simulink model "QuadModelv"  (R2022a)
settings: Solver=ode4  StartTime=0.0  StopTime=inf  FixedStep=0.001  RelTol=1e-3
PreLoadFcn:
  | filepath  = fileparts(get_param(bdroot, 'FileName'));
  | cd(filepath);
InitFcn:
  | Init
values from neighbouring files (symbols this model uses):
  ModelFailEnable = 0    [Init.m]
  ModelInit_RPM = 0    [Init.m]
  ModelParam_BattHoverMinutes = 18    [Init.m]
  ModelParam_BattHoverThr = 0.609    [Init.m]
  ModelParam_envAltitude = -50    [Init.m]
  ModelParam_GPSEphFinal = 0.3    [Init.m]
  ModelParam_GPSEpvFinal = 0.4    [Init.m]
  ModelParam_GPSFix3DFix = 3    [Init.m]
  ModelParam_GPSSatsVisible = 10    [Init.m]
  ModelParam_motorCr = 842.1    [Init.m]
  ModelParam_motorJm = 0.0001287    [Init.m]
  ModelParam_motorMinThr = 0.05    [Init.m]
  ModelParam_motorT = 0.0214    [Init.m]
  ModelParam_motorWb = 22.83    [Init.m]
  ModelParam_noiseGPSSampTime = 0.2    [Init.m]
  ModelParam_noisePowerOffGainAccel = 0.04    [Init.m]
  ModelParam_noisePowerOffGainAccelZ = 0.03    [Init.m]
  ModelParam_noisePowerOffGainGyro = 0.02    [Init.m]
  ModelParam_noisePowerOffGainGyroZ = 0.025    [Init.m]
  ModelParam_noisePowerOffGainMag = 0.02    [Init.m]
  ModelParam_noisePowerOffGainMagZ = 0.035    [Init.m]
  ModelParam_noisePowerOnGainAccel = 0.8    [Init.m]
  ModelParam_noisePowerOnGainAccelZ = 4.5    [Init.m]
  ModelParam_noisePowerOnGainGyro = 2    [Init.m]
  ModelParam_noisePowerOnGainGyroZ = 1    [Init.m]
  ModelParam_noisePowerOnGainMag = 0.025    [Init.m]
  ModelParam_noisePowerOnGainMagZ = 0.05    [Init.m]
  ModelParam_rotorCm = 2.783e-07    [Init.m]
  ModelParam_rotorCt = 1.681e-05    [Init.m]
  ModelParam_uavCCm = [0.0035 0.0039 0.0034]    [Init.m]
  ModelParam_uavCd = 0.055    [Init.m]
  ModelParam_uavDearo = 0.12    [Init.m]
  ModelParam_uavJ = [ModelParam_uavJxx,0,0;0,ModelParam_uavJyy,0;0,0,ModelParam_uavJzz]    [Init.m]
  ModelParam_uavMass = 1.515    [Init.m]
  ModelParam_uavMotNumbs = int8(4)    [Init.m]
  ModelParam_uavR = 0.225    [Init.m]
  ModelParam_uavType = int8(3)    [Init.m]
undefined symbols (not defined in the file or in its folder): d_i, Earth, h_i, ModelParam_GPSEpvInitial, ModelParam_GPSEpvTimeConstant, Newton, Raphson, WGS84
libraries: simulink x9, QuadModelLib x7, sharedtransform x3, aerolibtransform2 x2, sharedutil x2, aerolibutil x2, aerolibasang x2, shared6dof x1, aerolibatmos2 x1, aerolibconvert2 x1, aerolibobsolete x1
(part 3 of 3)

== matlab function QuadModelv/Force and Moment Model/Ground Model ==
  settings: updateMethod=DISCRETE
  data: mg input; wb input; Xe input; F1 output; Ve input; M1 output; Quet input; terrainZ input; landed output; takeoff output
function [F1,M1,landed,takeoff] = fcn(mg,wb,Xe,Ve,Quet,terrainZ)
% This is a ground model that can provides reaction force and reaction torque

% persistent z0;
% if isempty(z0)
%      z0=0;
% end

persistent takeoffFlag;
if isempty(takeoffFlag)
     takeoffFlag=int8(0);
end

persistent landFlag;
if isempty(landFlag)
     landFlag=int8(1);
end

z=Xe(3)-terrainZ;

if (z<-0.3)&&(Ve(3)<-0.1)&&(takeoffFlag<0.5)
    takeoffFlag=int8(1);
    landFlag=int8(0);
end

if (z>-0.05)&&(Ve(3)>0.1)&&(landFlag<0.5)
    landFlag=int8(1);
    takeoffFlag=int8(0);
end

takeoff = takeoffFlag;
landed = landFlag;


F1=[0;0;0];
M1=[0;0;0];

if z>=0
%     if z>=0.3
%         if Ve(3)>=5
%             F1(3)=-mg(3)-1000*Ve(3);
%         else
%             F1(3)=-mg(3)-500*z-100*Ve(3);  
%         end
%     elseif z>=0.1
%         if Ve(3)>=2
%             F1(3)=-mg(3)-100*Ve(3);
%         else
%             F1(3)=-mg(3)-50*z-100*Ve(3);  
%         end
%     else
%          if Ve(3)>=1
%             F1(3)=-mg(3)-50*Ve(3);
%         else
%             F1(3)=-mg(3)-5*z-50*Ve(3);  
%         end       
%     end
    if z<0.05
        F1(3)=-mg(3)-10*Ve(3); 
    elseif z<0.1
        F1(3)=-mg(3)-0.5*z-20*Ve(3); 
    else
        F1(3)=-mg(3)-1*z-50*Ve(3); 
    end

    F1(1)=-50*Ve(1);
    F1(2)=-50*Ve(2);
    
%     if ~(isnan(Quet(2))||isnan(Quet(3))||isnan(Quet(4)))
%         M1=-200*[Quet(2);Quet(3);Quet(4)]-10*wb;
%     end
    
    M1=-20*[Quet(2);Quet(3);Quet(4)]-5*wb;
    M1 = M1 * abs(mg(3))*0.0333;
end

== matlab function QuadModelv/Battery FaultModel/MATLAB Function ==
  data: load input; time input; EffRatio output; hover_time input; hover_thr input; motorNumbs input; cell_voltage output; isUseCustomHovTime input; CustomHovTime input; isPowOff input; isLowVoltage input; remainVoltageRatio input; islowCapacity input; remainCapacityRatio input; remCapacity output
function [EffRatio, cell_voltage,remCapacity]= LiPo(load,time,hover_time,hover_thr,motorNumbs,isUseCustomHovTime,CustomHovTime,isPowOff,isLowVoltage,remainVoltageRatio,islowCapacity,remainCapacityRatio)
%% battery model
%================================Constants=================================

delta_t = 0.01;
%max_current = 5.500;                % maximum current per motor             (A)
%aux_current = 0.100;                % current of auxillary components       (A)        
%capacity = 1.000;                   % LiPo current capacity                 (Ah)                                 
%cells = 2;                          % LiPo cell count

%==========================================================================

persistent discharge;
if isempty(discharge)
    discharge = 0;
end

persistent startTime;
if isempty(startTime)
    startTime = 0;
end

persistent reset;
if isempty(reset)
    reset = 0;
end

discharge_capacity=0;

% 低电量故障
if islowCapacity
   hover_time = hover_time*remainCapacityRatio(1);
   isUseCustomHovTime=false;
end


if ~isUseCustomHovTime 
    capacity=1;
    
    if hover_time<0.01
        hover_time=0.01;
    end
    
    hover_current=1/(hover_time*1.4/60);
    current=0;
    for i=1:motorNumbs
        current=current+hover_current*(load(i)/hover_thr)^2;
    end
    aux_current=0.5;
    %current = sum(hover_current .* (load/hover_thr).^2) + aux_current;
    current =(current+aux_current)/double(motorNumbs);
    discharge = current * (delta_t / 3600) + discharge;
    discharge_capacity = discharge / capacity;    
end




%如果启用电池模型且使用自定义续航时间
if isUseCustomHovTime
      hover_time=CustomHovTime(1)*1.4*60;
      if reset<0.5
         startTime=time;
         reset=1;
      end
      if hover_time<0.01
          hover_time=0.01;
      end
     discharge_capacity=(time-startTime)/hover_time;
else
    %使用默认的续航算法
    reset=0;
end


if discharge_capacity<0
    discharge_capacity=0;
end
if discharge_capacity>1
    discharge_capacity=1;
end


%电量与电压的曲线
if (0 <= discharge_capacity) && (discharge_capacity <=0.20)
    cell_voltage = -14.029*discharge_capacity^3 + 16.975*discharge_capacity^2 - 5.3339*discharge_capacity + 4.2;
elseif (0.20 < discharge_capacity) && (discharge_capacity < 0.70)
    cell_voltage = -0.2*discharge_capacity + 3.74;
else
    cell_voltage = -48*discharge_capacity^3 + 89.6*discharge_capacity^2 - 55.08*discharge_capacity + 14.716;
end

if cell_voltage < 0.5
    cell_voltage = 0;
end

% 电池失效故障
if isPowOff
     cell_voltage = 0; 
end

% 低电压故障
if isLowVoltage
    if remainVoltageRatio(1)>1
        remainVoltageRatio(1)=1;
    elseif remainVoltageRatio(1)<0
        remainVoltageRatio(1)=0;
    end
     cell_voltage = remainVoltageRatio(1)*4.2;
end


%如果电池模型未启用，续航为无穷久，同时各个全局变量归零
if ~isUseCustomHovTime&&~isPowOff&&~isLowVoltage&&~islowCapacity
    cell_voltage=4.2;
    discharge = 0;
    startTime = 0;
    reset = 0;
end

%效率矩阵
EffRatio=cell_voltage/4.2;
remCapacity=1-discharge_capacity;
%==========================================================================

== matlab function QuadModelv/LogSelectModel/MATLAB Function ==
  data: FaultIDs input; y output; D123450 input; D123451 input; D123452 input; unused input; unused90 input; unused91 input; D123456 input; unused92 input; unused93 input; D123459 input; unused94 input; unused95 input; unused96 input; unused97 input; D123544 input; D123545 input; D123546 input; D123547 input; D123548 input
function y = fcn(FaultIDs,D123450,D123451,D123452,~,~,~,D123456,~,~,D123459,~,~,~,~,D123544,D123545,D123546,D123547,D123548)

y = zeros(23,1);

FaultNum = 0;
for i = 1:8
    if FaultIDs(i)~=0
        FaultNum = FaultNum + 1;
    end
end


if FaultNum == 1
    if FaultIDs(1) == 123450|| FaultIDs(1) == 123549
        for i = 1:8
            y(i) = D123450(i);
        end
    elseif FaultIDs(1) == 123451
        for i = 1:8
            y(i) = D123451(i);
        end
    elseif FaultIDs(1) == 123452 || FaultIDs(1) == 123453 || FaultIDs(1) == 123454 || FaultIDs(1) == 123455
        for i = 1:2
            y(i) = D123452(i);
        end
    elseif FaultIDs(1) == 123456 || FaultIDs(1) == 123457 || FaultIDs(1) == 123458
        for i = 1:4
            y(i) = D123456(i);
        end
    elseif FaultIDs(1) == 123459 || FaultIDs(1) == 123540 || FaultIDs(1) == 123541 || FaultIDs(1) == 123542 || FaultIDs(1) == 123543
        for i = 1:6
            y(i) = D123459(i);
        end
    elseif FaultIDs(1) == 123544
        for i = 1:3
            y(i) = D123544(i);
        end
    elseif FaultIDs(1) == 123545
        for i = 1:3
            y(i) = D123545(i);
        end
    elseif FaultIDs(1) == 123546
        for i = 1:3
            y(i) = D123546(i);
        end
    elseif FaultIDs(1) == 123547
        y(1) = D123547(1);
    elseif FaultIDs(1) == 123548
        for i = 1:3
            y(i) = D123548(i);
        end
    end
end

if FaultNum == 2
    if FaultIDs(1) == 123450|| FaultIDs(1) == 123549
        for i = 1:8
            y(i) = D123450(i);
        end
        if FaultIDs(2) == 123451
            j = 1;
            for i = 9:16
                y(i) = D123451(j);
                j = j + 1;
            end
        elseif FaultIDs(2) == 123452 || FaultIDs(2) == 123453 || FaultIDs(2) == 123454 || FaultIDs(1) == 123455
            j = 1;
            for i = 9:10
                y(i) = D123452(j);
                j = j + 1;
            end
        elseif FaultIDs(2) == 123456 || FaultIDs(2) == 123457 || FaultIDs(2) == 123458
            j = 1;
            for i = 9:12
                y(i) = D123456(j);
                j = j + 1;
            end
        elseif FaultIDs(2) == 123459 || FaultIDs(2) == 123540 || FaultIDs(2) == 123541 || FaultIDs(2) == 123542 || FaultIDs(2) == 123543
            j = 1;
            for i = 9:14
                y(i) = D123459(j);
                j = j + 1;
            end
        elseif FaultIDs(2) == 123544
            j = 1;
            for i = 9:11
                y(i) = D123544(j);
                j = j + 1;
            end
        elseif FaultIDs(2) == 123545
            j = 1;
            for i = 9:11
                y(i) = D123545(j);
                j = j + 1;
            end
        elseif FaultIDs(2) == 123546
            j = 1;
            for i = 9:11
                y(i) = D123546(j);
                j = j + 1;
            end
        elseif FaultIDs(2) == 123547
            y(9) = D123547;
        elseif FaultIDs(2) == 123548
            j = 1;
            for i = 9:11
                y(i) = D123548(j);
                j = j + 1;
            end
        end
    elseif FaultIDs(1) == 123451
        for i = 1:8
            y(i) = D123451(i);
        end
        if FaultIDs(2) == 123450|| FaultIDs(2) == 123549
            j = 1;
            for i = 9:16
                y(i) = D123450(j);
                j = j + 1;
            end
        elseif FaultIDs(2) == 123452 || FaultIDs(2) == 123453 || FaultIDs(2) == 123454 || FaultIDs(1) == 123455
            j = 1;
            for i = 9:10
                y(i) = D123452(j);
                j = j + 1;
            end
        elseif FaultIDs(2) == 123456 || FaultIDs(2) == 123457 || FaultIDs(2) == 123458
            j = 1;
            for i = 9:12
                y(i) = D123456(j);
                j = j + 1;
            end
        elseif FaultIDs(2) == 123459 || FaultIDs(2) == 123540 || FaultIDs(2) == 123541 || FaultIDs(2) == 123542 || FaultIDs(2) == 123543
            j = 1;
            for i = 9:14
                y(i) = D123459(j);
                j = j + 1;
            end
        elseif FaultIDs(2) == 123544
            j = 1;
            for i = 9:11
                y(i) = D123544(j);
                j = j + 1;
            end
        elseif FaultIDs(2) == 123545
            j = 1;
            for i = 9:11
                y(i) = D123545(j);
                j = j + 1;
            end
        elseif FaultIDs(2) == 123546
            j = 1;
            for i = 9:11
                y(i) = D123546(j);
                j = j + 1;
            end
        elseif FaultIDs(2) == 123547
            y(9) = D123547;
        elseif FaultIDs(2) == 123548
            j = 1;
            for i = 9:11
                y(i) = D123548(j);
                j = j + 1;
            end
        end
    elseif FaultIDs(1) == 123452 || FaultIDs(1) == 123453 || FaultIDs(1) == 123454 || FaultIDs(1) == 123455
        for i = 1:2
            y(i) = D123452(i);
        end
        if FaultIDs(2) == 123450|| FaultIDs(2) == 123549
            j = 1;
            for i = 3:10
                y(i) = D123450(j);
                j = j + 1;
            end
        elseif FaultIDs(2) == 123451
            j = 1;
            for i = 3:10
                y(i) = D123451(j);
                j = j + 1;
            end
        elseif FaultIDs(2) == 123456 || FaultIDs(2) == 123457 || FaultIDs(2) == 123458
            j = 1;
            for i = 3:6
                y(i) = D123456(j);
                j = j + 1;
            end
        elseif FaultIDs(2) == 123459 || FaultIDs(2) == 123540 || FaultIDs(2) == 123541 || FaultIDs(2) == 123542 || FaultIDs(2) == 123543
            j = 1;
            for i = 3:8
                y(i) = D123459(j);
                j = j + 1;
            end
        elseif FaultIDs(2) == 123544
            j = 1;
            for i = 3:5
                y(i) = D123544(j);
                j = j + 1;
            end
        elseif FaultIDs(2) == 123545
            j = 1;
            for i = 3:5
                y(i) = D123545(j);
                j = j + 1;
            end
        elseif FaultIDs(2) == 123546
            j  = 1;
            for i = 3:5
                y(i) = D123546(j);
                j = j + 1;
            end
        elseif FaultIDs(2) == 123547
            y(3) = D123547;
        elseif FaultIDs(2) == 123548
            j = 1;
            for i = 3:5
                y(i) = D123548(j);
                j = j + 1;
            end
        end
    elseif FaultIDs(1) == 123456 || FaultIDs(1) == 123457 || FaultIDs(1) == 123458
        for i = 1:4
            y(i) = D123456(i);
        end
        if FaultIDs(2) == 123450|| FaultIDs(2) == 123549
            j = 1;
            for i = 5:12
                y(i) = D123450(j);
                j = j + 1;
            end
        elseif FaultIDs(2) == 123451
            j = 1;
            for i = 5:12
                y(i) = D123451(j);
                j = j + 1;
            end
        elseif FaultIDs(2) == 123452 || FaultIDs(2) == 123453 || FaultIDs(2) == 123454 || FaultIDs(2) == 123455
            j = 1;
            for i = 5:6
                y(i) = D123452(j);
                j = j + 1;
            end
        elseif FaultIDs(2) == 123459 || FaultIDs(2) == 123540 || FaultIDs(2) == 123541 || FaultIDs(2) == 123542 || FaultIDs(2) == 123543
            j = 1;
            for i = 5:10
                y(i) = D123459(j);
                j = j + 1;
            end
        elseif FaultIDs(2) == 123544
            j = 1;
            for i = 5:7
                y(i) = D123544(j);
                j = j + 1;
            end
        elseif FaultIDs(2) == 123545
            j = 1;
            for i = 5:7
                y(i) = D123545(j);
                j = j + 1;
            end
        elseif FaultIDs(2) == 123546
            j = 1;
            for i = 5:7
                y(i) = D123546(j);
                j = j + 1;
            end
        elseif FaultIDs(2) == 123547
            y(5) = D123547;
        elseif FaultIDs(2) == 123548
            j = 1;
            for i = 5:7
                y(i) = D123548(j);
                j = j + 1;
            end
        end
    elseif FaultIDs(1) == 123459 || FaultIDs(1) == 123540 || FaultIDs(1) == 123541 || FaultIDs(1) == 123542 || FaultIDs(1) == 123543
        for i = 1:6
            y(i) = D123459(i);
        end
        if FaultIDs(2) == 123450|| FaultIDs(2) == 123549
            j = 1;
            for i = 7:14
                y(i) = D123450(j);
                j = j + 1;
            end
        elseif FaultIDs(2) == 123451
            j = 1;
            for i = 7:14
                y(i) = D123451(j);
                j = j + 1;
            end
        elseif FaultIDs(2) == 123452 || FaultIDs(2) == 123453 || FaultIDs(2) == 123454 || FaultIDs(2) == 123455
            j = 1;
            for i = 7:8
                y(i) = D123452(j);
                j = j + 1;
            end
        elseif FaultIDs(2) == 123456 || FaultIDs(2) == 123457 || FaultIDs(2) == 123458
            j = 1;
            for i = 7:12
                y(i) = D123456(j);
                j = j + 1;
            end
        elseif FaultIDs(2) == 123544
            j = 1;
            for i = 7:9
                y(i) = D123544(j);
                j = j + 1;
            end
        elseif FaultIDs(2) == 123545
            j = 1;
            for i = 7:9
                y(i) = D123545(j);
                j = j + 1;
            end
        elseif FaultIDs(2) == 123546
            j = 1;
            for i = 7:9
                y(i) = D123546(j);
                j = j + 1;
            end
        elseif FaultIDs(2) == 123547
            y(7) = D123547;
        elseif FaultIDs(2) == 123548
            j = 1;
            for i = 7:9
                y(i) = D123548(j);
                j = j + 1;
            end
        end
    elseif FaultIDs(1) == 123544
        for i = 1:3
            y(i) = D123544(i);
        end
        if FaultIDs(2) == 123450|| FaultIDs(2) == 123549
            j = 1;
            for i = 4:11
                y(i) = D123450(j);
                j = j + 1;
            end
        elseif FaultIDs(2) == 123451
            j = 1;
            for i = 4:11
                y(i) = D123451(j);
                j = j + 1;
            end
        elseif FaultIDs(2) == 123452 || FaultIDs(2) == 123453 || FaultIDs(2) == 123454 || FaultIDs(2) == 123455
            j = 1;
            for i = 4:5
                y(i) = D123452(j);
                j = j + 1;
            end
        elseif FaultIDs(2) == 123456 || FaultIDs(2) == 123457 || FaultIDs(2) == 123458
            j = 1;
            for i = 4:9
                y(i) = D123456(j);
                j = j + 1;
            end
        elseif FaultIDs(2) == 123459 || FaultIDs(2) == 123540 || FaultIDs(2) == 123541 || FaultIDs(2) == 123542 || FaultIDs(2) == 123543
            j = 1;
            for i = 4:9
                y(i) = D123459(j);
                j = j + 1;
            end
        elseif FaultIDs(2) == 123545
            j = 1;
            for i = 4:6
                y(i) = D123545(j);
                j = j + 1;
            end
        elseif FaultIDs(2) == 123546
            j = 1;
            for i = 4:6
                y(i) = D123546(j);
                j = j + 1;
            end
        elseif FaultIDs(2) == 123547
            y(4) = D123547;
        elseif FaultIDs(2) == 123548
            j = 1;
            for i = 4:6
                y(i) = D123548(j);
                j = j + 1;
            end
        end
    elseif FaultIDs(1) == 123545
        for i = 1:3
            y(i) = D123545(i);
        end
        if FaultIDs(2) == 123450|| FaultIDs(2) == 123549
            j = 1;
            for i = 4:11
                y(i) = D123450(j);
                j = j + 1;
            end
        elseif FaultIDs(2) == 123451
            j = 1;
            for i = 4:11
                y(i) = D123451(j);
                j = j + 1;
            end
        elseif FaultIDs(2) == 123452 || FaultIDs(2) == 123453 || FaultIDs(2) == 123454 || FaultIDs(2) == 123455
            j = 1;
            for i = 4:5
                y(i) = D123452(j);
                j = j + 1;
            end
        elseif FaultIDs(2) == 123456 || FaultIDs(2) == 123457 || FaultIDs(2) == 123458
            j = 1;
            for i = 4:9
                y(i) = D123456(j);
                j = j + 1;
            end
        elseif FaultIDs(2) == 123459 || FaultIDs(2) == 123540 || FaultIDs(2) == 123541 || FaultIDs(2) == 123542 || FaultIDs(2) == 123543
            j = 1;
            for i = 4:9
                y(i) = D123459(j);
                j = j + 1;
            end
        elseif FaultIDs(2) == 123544
            j = 1;
            for i = 4:6
                y(i) = D123544(j);
                j = j + 1;
            end
        elseif FaultIDs(2) == 123546
            j = 1;
            for i = 4:6
                y(i) = D123546(j);
                j = j + 1;
            end
        elseif FaultIDs(2) == 123547
            y(4) = D123547;
        elseif FaultIDs(2) == 123548
            j = 1;
            for i = 4:6
                y(i) = D123548(j);
                j = j + 1;
            end
        end
    elseif FaultIDs(1) == 123546
        for i = 1:3
            y(i) = D123545(i);
        end
        if FaultIDs(2) == 123450|| FaultIDs(2) == 123549
            j = 1;
            for i = 4:11
                y(i) = D123450(j);
                j = j + 1;
            end
        elseif FaultIDs(2) == 123451
            j = 1;
            for i = 4:11
                y(i) = D123451(j);
                j = j + 1;
            end
        elseif FaultIDs(2) == 123452 || FaultIDs(2) == 123453 || FaultIDs(2) == 123454 || FaultIDs(2) == 123455
            j = 1;
            for i = 4:5
                y(i) = D123452(j);
                j = j + 1;
            end
        elseif FaultIDs(2) == 123456 || FaultIDs(2) == 123457 || FaultIDs(2) == 123458
            j = 1;
            for i = 4:9
                y(i) = D123456(j);
                j = j + 1;
            end
        elseif FaultIDs(2) == 123459 || FaultIDs(2) == 123540 || FaultIDs(2) == 123541 || FaultIDs(2) == 123542 || FaultIDs(2) == 123543
            j = 1;
            for i = 4:9
                y(i) = D123459(j);
                j = j + 1;
            end
        elseif FaultIDs(2) == 123544
            j = 1;
            for i = 4:6
                y(i) = D123544(j);
                j = j + 1;
            end
        elseif FaultIDs(2) == 123545
            j = 1;
            for i = 4:6
                y(i) = D123545(j);
                j = j + 1;
            end
        elseif FaultIDs(2) == 123547
            y(4) = D123547;
        elseif FaultIDs(2) == 123548
            j = 1;
            for i = 4:6
                y(i) = D123548(j);
                j = j + 1;
            end
        end
    elseif FaultIDs(1) == 123547
        y(1) = D123547(1);
        if FaultIDs(2) == 123450|| FaultIDs(2) == 123549
            j = 1;
            for i = 2:9
                y(i) = D123450(j);
                j = j + 1;
            end
        elseif FaultIDs(2) == 123451
            j = 1;
            for i = 2:9
                y(i) = D123451(j);
                j = j + 1;
            end
        elseif FaultIDs(2) == 123452 || FaultIDs(2) == 123453 || FaultIDs(2) == 123454 || FaultIDs(2) == 123455
            j = 1;
            for i = 2:3
                y(i) = D123452(j);
                j = j + 1;
            end
        elseif FaultIDs(2) == 123456 || FaultIDs(2) == 123457 || FaultIDs(2) == 123458
            j = 1;
            for i = 2:7
                y(i) = D123456(j);
                j = j + 1;
            end
        elseif FaultIDs(2) == 123459 || FaultIDs(2) == 123540 || FaultIDs(2) == 123541 || FaultIDs(2) == 123542 || FaultIDs(2) == 123543
            j = 1;
            for i = 2:7
                y(i) = D123459(j);
                j = j + 1;
            end
        elseif FaultIDs(2) == 123544
            j = 1;
            for i = 2:4
                y(i) = D123544(j);
                j = j + 1;
            end
        elseif FaultIDs(2) == 123545
            j = 1;
            for i = 2:4
                y(i) = D123545(j);
                j = j + 1;
            end
        elseif FaultIDs(2) == 123546
            j = 1;
           for i = 2:4
                y(i) = D123546(j);
                j = j + 1;
            end
        elseif FaultIDs(2) == 123548
            j = 1;
            for i = 2:4
                y(i) = D123548(j);
                j = j + 1;
            end
        end
    elseif FaultIDs(1) == 123548
        for i = 1:3
            y(i) = D123548(i);
        end
        if FaultIDs(2) == 123450|| FaultIDs(2) == 123549
            j = 1;
            for i = 4:11
                y(i) = D123450(j);
                j = j + 1;
            end
        elseif FaultIDs(2) == 123451
            j = 1;
            for i = 4:11
                y(i) = D123451(j);
                j = j + 1;
            end
        elseif FaultIDs(2) == 123452 || FaultIDs(2) == 123453 || FaultIDs(2) == 123454 || FaultIDs(2) == 123455
            j = 1;
            for i = 4:5
                y(i) = D123452(j);
                j = j + 1;
            end
        elseif FaultIDs(2) == 123456 || FaultIDs(2) == 123457 || FaultIDs(2) == 123458
            j = 1;
            for i = 4:9
                y(i) = D123456(j);
                j = j + 1;
            end
        elseif FaultIDs(2) == 123459 || FaultIDs(2) == 123540 || FaultIDs(2) == 123541 || FaultIDs(2) == 123542 || FaultIDs(2) == 123543
            j = 1;
            for i = 4:9
                y(i) = D123459(j);
                j = j + 1;
            end
        elseif FaultIDs(2) == 123544
            j = 1;
            for i = 4:6
                y(i) = D123544(j);
                j = j + 1;
            end
        elseif FaultIDs(2) == 123545
            j = 1;
            for i = 4:6
                y(i) = D123545(j);
                j = j + 1;
            end
        elseif FaultIDs(2) == 123547
            y(4) = D123547;
        elseif FaultIDs(2) == 123546
            j = 1;
            for i = 4:6
                y(i) = D123546(j);
                j = j + 1;
            end
        end
    end
end

if FaultNum >= 3
    if any(find(FaultIDs==123450|FaultIDs==123549))&&any(find(FaultIDs==123452|FaultIDs==123453|FaultIDs==123454|FaultIDs==123455))&&any(find(FaultIDs==123456|FaultIDs==123457|FaultIDs==123458))
        for i = 1:8
            y(i) = D123450(i);
        end
        j = 1;
        for i = 9:10
            y(i) = D123452(j);
            j = j + 1;
        end
        k = 1;
        for i = 11:14
            y(i) = D123456(k);
            k = k + 1;
        end
    elseif any(find(FaultIDs==123450|FaultIDs==123549))&&any(find(FaultIDs==123452|FaultIDs==123453|FaultIDs==123454|FaultIDs==123455))&&any(find(FaultIDs==123459|FaultIDs==123540|FaultIDs==123541|FaultIDs==123542|FaultIDs==123543))
        for i = 1:8
            y(i) = D123450(i);
        end
        j = 1;
        for i = 9:10
            y(i) = D123452(j);
            j = j + 1;
        end
        k = 1;
        for i = 11:16
            y(i) = D123459(k);
            k = k + 1;
        end
    elseif any(find(FaultIDs==123450|FaultIDs==123549))&&any(find(FaultIDs==123452|FaultIDs==123453|FaultIDs==123454|FaultIDs==123455))&&any(find(FaultIDs==123544|FaultIDs==123545|FaultIDs==123546|FaultIDs==123548|FaultIDs==123547))
        for i = 1:8
            y(i) = D123450(i);
        end
        j = 1;
        for i = 9:10
            y(i) = D123452(j);
            j = j + 1;
        end
        k = 1;
        if any(find(FaultIDs==123544))
            for i = 11:13
                y(i) = D123544(k);
                k = k + 1;
            end
        elseif any(find(FaultIDs==123545))
            for i = 11:13
                y(i) = D123545(k);
                k = k + 1;
            end
        elseif any(find(FaultIDs==123546))
            for i = 11:13
                y(i) = D123546(k);
                k = k + 1;
            end
        elseif any(find(FaultIDs==123548))
            for i = 11:13
                y(i) = D123548(k);
                k = k + 1;
            end
        elseif any(find(FaultIDs==123547))
           y(11) = D123547;
        end
    elseif any(find(FaultIDs==123452|FaultIDs==123453|FaultIDs==123454|FaultIDs==123455))&&any(find(FaultIDs==123456|FaultIDs==123457|FaultIDs==123458))&&any(find(FaultIDs==123459|FaultIDs==123540|FaultIDs==123541|FaultIDs==123542|FaultIDs==123543))
        for i = 1:2
            y(i) = D123452(i);
        end
        j = 1;
        for i = 3:6
            y(i) = D123456(j);
            j = j + 1;
        end
        k = 1;
        for i = 7:12
            y(i) = D123459(k);
            k = k + 1;
        end
    elseif any(find(FaultIDs==123452|FaultIDs==123453|FaultIDs==123454|FaultIDs==123455))&&any(find(FaultIDs==123456|FaultIDs==123457|FaultIDs==123458))&&any(find(FaultIDs==123544|FaultIDs==123545|FaultIDs==123546|FaultIDs==123548|FaultIDs==123547))
        for i = 1:2
            y(i) = D123452(i);
        end
        j = 1;
        for i = 3:6
            y(i) = D123456(j);
            j = j + 1;
        end
        k = 1;
        if any(find(FaultIDs==123544))
            for i = 7:9
                y(i) = D123544(k);
                k = k + 1;
            end
        elseif any(find(FaultIDs==123545))
            for i = 7:9
                y(i) = D123545(k);
                k = k + 1;
            end
        elseif any(find(FaultIDs==123546))
            for i = 7:9
                y(i) = D123546(k);
                k = k + 1;
            end
        elseif any(find(FaultIDs==123548))
            for i = 7:9
                y(i) = D123548(k);
                k = k + 1;
            end
        elseif any(find(FaultIDs==123547))
           y(7) = D123547;
        end
    elseif any(find(FaultIDs==123456|FaultIDs==123457|FaultIDs==123458))&&any(find(FaultIDs==123544|FaultIDs==123545|FaultIDs==123546|FaultIDs==123548|FaultIDs==123547))&&any(find(FaultIDs==123459|FaultIDs==123540|FaultIDs==123541|FaultIDs==123542|FaultIDs==123543))
        for i = 1:4
            y(i) = D123456(i);
        end
        j = 1;
        for i = 5:10
            y(i) = D123459(j);
            j = j + 1;
        end
        k = 1;
        if any(find(FaultIDs==123544))
            for i = 11:13
                y(i) = D123544(k);
                k = k + 1;
            end
        elseif any(find(FaultIDs==123545))
            for i = 11:13
                y(i) = D123545(k);
                k = k + 1;
            end
        elseif any(find(FaultIDs==123546))
            for i = 11:13
                y(i) = D123546(k);
                k = k + 1;
            end
        elseif any(find(FaultIDs==123548))
            for i = 11:13
                y(i) = D123548(k);
                k = k + 1;
            end
        elseif any(find(FaultIDs==123547))
           y(11) = D123547;
        end
    elseif any(find(FaultIDs==123450|FaultIDs==123549))&&any(find(FaultIDs==123456|FaultIDs==123457|FaultIDs==123458))&&any(find(FaultIDs==123459|FaultIDs==123540|FaultIDs==123541|FaultIDs==123542|FaultIDs==123543))
        for i = 1:8
            y(i) = D123450(i);
        end
        j = 1;
        for i = 9:12
            y(i) = D123456(j);
            j = j + 1;
        end
        k = 1;
        for i = 13:18
            y(i) = D123459(k);
            k = k + 1;
        end
    elseif any(find(FaultIDs==123450|FaultIDs==123549))&&any(find(FaultIDs==123456|FaultIDs==123457|FaultIDs==123458))&&any(find(FaultIDs==123544|FaultIDs==123545|FaultIDs==123546|FaultIDs==123548|FaultIDs==123547))
        for i = 1:8
            y(i) = D123450(i);
        end
        j = 1;
        for i = 9:12
            y(i) = D123456(j);
            j = j + 1;
        end
        k = 1;
        if any(find(FaultIDs==123544))
            for i = 13:15
                y(i) = D123544(k);
                k = k + 1;
            end
        elseif any(find(FaultIDs==123545))
            for i = 13:15
                y(i) = D123545(k);
                k = k + 1;
            end
        elseif any(find(FaultIDs==123546))
            for i = 13:15
                y(i) = D123546(k);
                k = k + 1;
            end
        elseif any(find(FaultIDs==123548))
            for i = 13:15
                y(i) = D123548(k);
                k = k + 1;
            end
        elseif any(find(FaultIDs==123547))
           y(13) = D123547;
        end
    elseif any(find(FaultIDs==123450|FaultIDs==123549))&&any(find(FaultIDs==123459|FaultIDs==123540|FaultIDs==123541|FaultIDs==123542|FaultIDs==123543))&&any(find(FaultIDs==123544|FaultIDs==123545|FaultIDs==123546|FaultIDs==123548|FaultIDs==123547))
        for i = 1:8
            y(i) = D123450(i);
        end
        j = 1;
        for i = 9:14
            y(i) = D123459(j);
            j = j + 1;
        end
        k = 1;
        if any(find(FaultIDs==123544))
            for i = 15:17
                y(i) = D123544(k);
                k = k + 1;
            end
        elseif any(find(FaultIDs==123545))
            for i = 15:17
                y(i) = D123545(k);
                k = k + 1;
            end
        elseif any(find(FaultIDs==123546))
            for i = 15:17
                y(i) = D123546(k);
                k = k + 1;
            end
        elseif any(find(FaultIDs==123548))
            for i = 15:17
                y(i) = D123548(k);
                k = k + 1;
            end
        elseif any(find(FaultIDs==123547))
           y(15) = D123547;
        end
    elseif any(find(FaultIDs==123452|FaultIDs==123453|FaultIDs==123454|FaultIDs==123455))&&any(find(FaultIDs==123459|FaultIDs==123540|FaultIDs==123541|FaultIDs==123542|FaultIDs==123543))&&any(find(FaultIDs==123544|FaultIDs==123545|FaultIDs==123546|FaultIDs==123548|FaultIDs==123547))
        for i = 1:2
            y(i) = D123452(i);
        end
        j = 1;
        for i = 3:8
            y(i) = D123459(j);
            j = j + 1;
        end
        k = 1;
        if any(find(FaultIDs==123544))
            for i = 8:10
                y(i) = D123544(k);
                k = k + 1;
            end
        elseif any(find(FaultIDs==123545))
            for i = 8:10
                y(i) = D123545(k);
                k = k + 1;
            end
        elseif any(find(FaultIDs==123546))
            for i = 8:10
                y(i) = D123546(k);
                k = k + 1;
            end
        elseif any(find(FaultIDs==123548))
            for i = 8:10
                y(i) = D123548(k);
                k = k + 1;
            end
        elseif any(find(FaultIDs==123547))
           y(8) = D123547;
        end
    elseif any(find(FaultIDs==123450|FaultIDs==123549))&&any(find(FaultIDs==123452|FaultIDs==123453|FaultIDs==123454|FaultIDs==123455))
        for i = 1:8
            y(i) = D123450(i);
        end
        j = 1;
        for i = 9:10
            y(i) = D123452(j);
            j = j + 1;
        end
    elseif any(find(FaultIDs==123450|FaultIDs==123549))&&any(find(FaultIDs==123456|FaultIDs==123457|FaultIDs==123458))
        for i = 1:8
            y(i) = D123450(i);
        end
        j = 1;
        for i = 9:12
            y(i) = D123456(j);
            j = j + 1;
        end
    elseif any(find(FaultIDs==123450|FaultIDs==123549))&&any(find(FaultIDs==123459|FaultIDs==123540|FaultIDs==123541|FaultIDs==123542|FaultIDs==123543))
        for i = 1:8
            y(i) = D123450(i);
        end
        j = 1;
        for i = 9:14
            y(i) = D123459(j);
            j = j + 1;
        end
    elseif any(find(FaultIDs==123452|FaultIDs==123453|FaultIDs==123454|FaultIDs==123455))&&any(find(FaultIDs==123456|FaultIDs==123457|FaultIDs==123458))
        for i = 1:2
            y(i) = D123452(i);
        end
        j = 1;
        for i = 3:6
            y(i) = D123456(j);
            j = j + 1;
        end
    elseif any(find(FaultIDs==123452|FaultIDs==123453|FaultIDs==123454|FaultIDs==123455))&&any(find(FaultIDs==123459|FaultIDs==123540|FaultIDs==123541|FaultIDs==123542|FaultIDs==123543))
        for i = 1:2
            y(i) = D123452(i);
        end
        j = 1;
        for i = 3:8
            y(i) = D123459(j);
            j = j + 1;
        end
    elseif any(find(FaultIDs==123456|FaultIDs==123457|FaultIDs==123458))&&any(find(FaultIDs==123459|FaultIDs==123540|FaultIDs==123541|FaultIDs==123542|FaultIDs==123543))
        for i = 1:4
            y(i) = D123456(i);
        end
        j = 1;
        for i = 5:10
            y(i) = D123459(j);
            j = j + 1;
        end
    else
        for i = 1:8
            y(i) = D123450(i);
        end
        j = 1;
        for i = 9:10
            y(i) = D123452(j);
            j = j + 1;
        end
        c = 1;
        for i = 10:13
            y(i) = D123456(c);
            c = c + 1;
        end
        q = 1;
        for i = 14:19
            y(i) = D123459(q);
            q = q + 1;
        end
        k = 1;
        if any(find(FaultIDs==123544))
            for i = 20:22
                y(i) = D123544(k);
                k = k + 1;
            end
        elseif any(find(FaultIDs==123545))
            for i = 20:22
                y(i) = D123545(k);
                k = k + 1;
            end
        elseif any(find(FaultIDs==123546))
            for i = 20:22
                y(i) = D123546(k);
                k = k + 1;
            end
        elseif any(find(FaultIDs==123548))
            for i = 20:22
                y(i) = D123548(k);
                k = k + 1;
            end
        elseif any(find(FaultIDs==123547))
           y(20) = D123547;
        end
    end
end
